simulink model "discreteSSmodel_check"  (R2016b)
settings: Solver=FixedStepDiscrete  StartTime=0.0  StopTime=50  FixedStep=0.05  RelTol=1e-3
values from neighbouring files (symbols this model uses):
  Ad = d_sys.A    [ControllerLQR.m]    (also in plotData.m)
  Bd = d_sys.B    [ControllerLQR.m]    (also in plotData.m)
  Cd = d_sys.C    [ControllerLQR.m]    (also in plotData.m)
  init_cond = [yaw_in yawd_in xb_in]    [plotData.m]
settings Model: Creator=himalkooverjee  LastModifiedBy=himalkooverjee

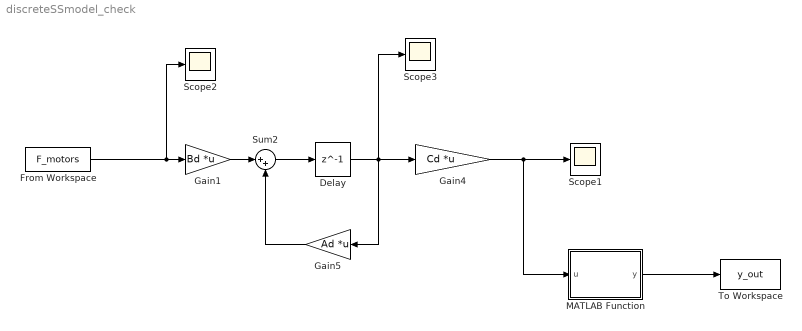
== system discreteSSmodel_check ==
  Delay : Delay  DelayLength=1  InitialCondition=init_cond
  From Workspace : FromWorkspace  VariableName=F_motors
  Gain1 : Gain  Gain=Bd  Multiplication=Matrix(K*u)
  Gain4 : Gain  Gain=Cd  Multiplication=Matrix(K*u)
  Gain5 : Gain  Gain=Ad  Multiplication=Matrix(K*u)
  MATLAB Function : MATLAB Function  TreatAsAtomicUnit=on
  Scope1 : Scope
  Scope2 : Scope
  Scope3 : Scope
  Sum2 : Sum  Inputs=|++
  To Workspace : ToWorkspace  VariableName=y_out  SaveFormat=Timeseries  SampleTime=-1
  wires:
  Delay/1 -> Scope3/1, Gain5/1, Gain4/1
  Gain4/1 -> MATLAB Function/1(u), Scope1/1
  Gain1/1 -> Sum2/1
  Gain5/1 -> Sum2/2
  Sum2/1 -> Delay/1
  From Workspace/1 -> Scope2/1, Gain1/1
  MATLAB Function/1(y) -> To Workspace/1

== matlab function discreteSSmodel_check/MATLAB Function ==
  data: u input; y output
function y = fcn(u)

u(1) = mod(u(1),2*pi)-pi;
% if u(1) > pi
%     u(1) = u(1) - 2*pi
% end
% if u(1) < -pi
%     u(1) = u(1) + 2*pi
% end


y = u;
